simulink model "master_1"  (Simulink 7.8)
settings: Solver=ode3  StartTime=0.0  StopTime=inf  RelTol=1e-3
libraries: xpcethercatlib x7, xpclib x2
settings Model: Creator=hareen  LastModifiedBy=KTmp  SimulationMode=external  BufferReuse=off
settings OptimizationCC: BlockReduction=off  OptimizeBlockIOStorage=off  BufferReuse=off  ExpressionFolding=off  LocalBlockOutputs=off
settings HardwareCC: ProdIntDivRoundTo=Zero  ProdEndianess=LittleEndian  ProdHWDeviceType=Generic->32-bit x86 compatible
settings RTWCC: SystemTargetFile=xpctarget.tlc  TemplateMakefile=xpc_default_tmf  Description=xPC Target  ProcessScript=xpctarget_make_rtw_hook  RTWCompilerOptimization=On
settings xpcTargetCC: TargetFcnLib=ansi_tfl_table_tmw.mat  TargetFunctionLibrary=XPC_BLAS  CodeExecutionProfiling=off  ParMdlRefBuildCompliant=on  ConcurrentExecutionCompliant=on  CombineSignalStateStructs=off  PortableWordSizes=off  xPCTaskExecutionProfile=off  xPCRL32EventNumber=5000  xPCLoadParamSetFile=off  xPCConcurrentTasks=off  xPCEnableSFAnimation=off

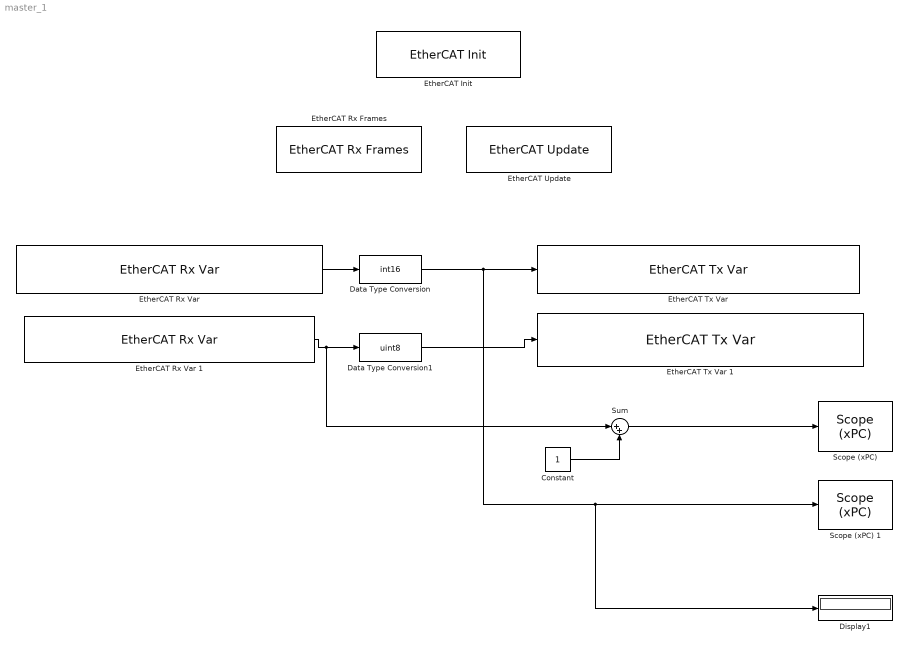
== system master_1 ==
  Constant : Constant
  Data Type Conversion : DataTypeConversion  OutDataTypeStr=int16
  Data Type Conversion1 : DataTypeConversion  OutDataTypeStr=uint8
  Display1 : Display
  "EtherCAT Init " : xpcethercatlib/EtherCAT Init   Priority=0  config_file='medulla_debug7.xml'  device_id=0  pci_bus=5  pci_slot=5  enaDC=off  errRptLevel=0  sample_time=-1
  "EtherCAT Rx Frames " : xpcethercatlib/EtherCAT Rx Frames   Priority=1  device_id=0  sample_time=0
  "EtherCAT Rx Var " : xpcethercatlib/EtherCAT Rx Var   Priority=2  sig_name=Box 1 (ATRIAS 2.1 EtherCAT Test (Medulla 1.5)).uControllerOutput.Encoder 0  sig_offset=224  sig_type=uint32  type_size=32  sig_dim=1  device_id=0  sample_time=0.010000
  EtherCAT Rx Var 1 : xpcethercatlib/EtherCAT Rx Var   Priority=2  sig_name=Box 1 (ATRIAS 2.1 EtherCAT Test (Medulla 1.5)).uControllerOutput.Timestep  sig_offset=208  sig_type=uint16  type_size=16  sig_dim=1  device_id=0  sample_time=0.010000
  "EtherCAT Tx Var " : xpcethercatlib/EtherCAT Tx Var   Priority=3  sig_name=Box 1 (ATRIAS 2.1 EtherCAT Test (Medulla 1.5)).uControllerInput.Motor Current  sig_offset=216  sig_type=int16  type_size=16  sig_dim=1  device_id=0  sample_time=0.01
  EtherCAT Tx Var 1 : xpcethercatlib/EtherCAT Tx Var   Priority=3  sig_name=Box 1 (ATRIAS 2.1 EtherCAT Test (Medulla 1.5)).uControllerInput.Command  sig_offset=208  sig_type=uint8  type_size=8  sig_dim=1  device_id=0  sample_time=0.01
  "EtherCAT Update " : xpcethercatlib/EtherCAT Update   Priority=4  device_id=0  task_id_list=[1]  task_rates=[10]  task_priorities=[0]
  "Scope (xPC) " : xpclib/Misc./Scope (xPC)   scopeno=1  scopetype=Target  autostart=on  viewmode=Numerical  formatstr='%15.6f'  grid=on  ylimits=[0,0]  nosamples=250  noprepostsamples=0  interleave=1  triggermode=FreeRun  triggersignal=1  triggerlevel=0.0  triggerslope=Either  triggerscope=1  triggersample=0  filename=data.dat  mode=Lazy  writesize=512  autorestart=off  dynamicfilemode=off  maxwritefilesize=512*1024^2
  Scope (xPC) 1 : xpclib/Misc./Scope (xPC)   scopeno=2  scopetype=Target  autostart=on  viewmode=Numerical  formatstr='%15.6f'  grid=on  ylimits=[0,0]  nosamples=250  noprepostsamples=0  interleave=1  triggermode=FreeRun  triggersignal=1  triggerlevel=0.0  triggerslope=Either  triggerscope=1  triggersample=0  filename=data.dat  mode=Lazy  writesize=512  autorestart=off  dynamicfilemode=off  maxwritefilesize=512*1024^2
  Sum : Sum  Inputs=|++
  wires:
  "EtherCAT Rx Var "/1 -> Data Type Conversion/1
  EtherCAT Rx Var 1/1 -> Data Type Conversion1/1, Sum/1
  Data Type Conversion/1 -> "EtherCAT Tx Var "/1, Scope (xPC) 1/1, Display1/1
  Data Type Conversion1/1 -> EtherCAT Tx Var 1/1
  Sum/1 -> "Scope (xPC) "/1
  Constant/1 -> Sum/2
